simulink model "efficiency_model"  (R2024b)
settings: Solver=VariableStepAuto  StartTime=0.0  StopTime=10.0  RelTol=1e-3
settings Model: Creator=marti  LastModifiedBy=marti

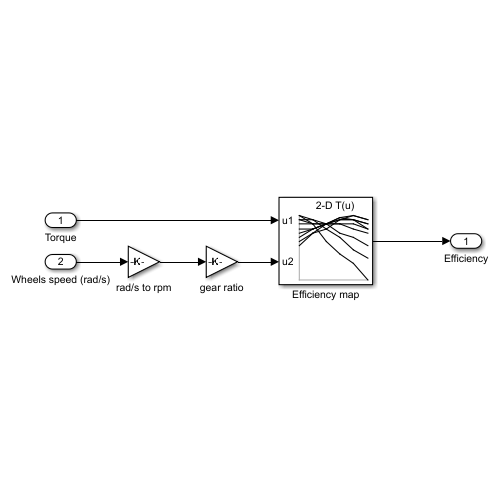
[thumbnail: Simulink's stored preview of the top-level diagram]
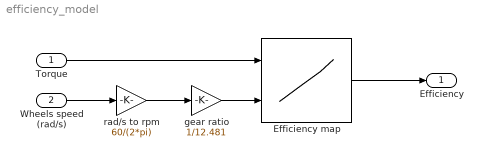
== system efficiency_model ==
  Torque : Inport
  Wheels speed (rad/s) : Inport  Port=2
  Efficiency map : Lookup_n-D  BreakpointsForDimension1=[0;5;10;15;20;25]  BreakpointsForDimension2=[2000;4000;6000;8000;10000;12000;14000;16000;18000;20000]  Table=[98 98 97 97 96 95 94 93 92 91;96 97 97 96 96 95 95 95 94 94;92 95 96 96 96 96 96 96 96 95;89 93 94 96 96 97 97 97.5 97.5 97;87 90 93 95 96 97 97 97 98 98;83 88 91 94 95 95 96 96 97 97]  InternalRulePriority=Speed  RndMeth=Simplest
      settings: InputPortMap=u0,u1
  gear ratio : Gain  Gain=1/12.481
  rad/s to rpm : Gain  Gain=60/(2*pi)
  Efficiency : Outport
  wires:
  Wheels speed (rad/s)/1 -> rad/s to rpm/1
  rad/s to rpm/1 -> gear ratio/1
  Torque/1 -> Efficiency map/1
  Efficiency map/1 -> Efficiency/1
  gear ratio/1 -> Efficiency map/2
